simulink model "Simulink_model"  (Simulink 7.9)
settings: Solver=ode45  StartTime=0.0  StopTime=2  RelTol=1e-3
PreLoadFcn:
  | %% パラメータ設定
  | Ra = 1;%アーマチュア抵抗[Ω]
  | La = 1e-5;%アーマチュアインダクタンス[H]
  | KT = 0.05;%トルク定数[N*m/A]
  | KE = KT;%逆起定数[V*s/rad]
  | %その他パラメータ
  | K = 0.5;%バネ定数[N*m*rad^-1*s]
  | D = 5e-5;%粘性摩擦[N*m*rad^-1*s^2]
  | L = 0.02;%無駄時間[s]
  | 
  | JM = 1e-4;%ロータ側のイナーシャ[kg*m^2]
  | JL = 0.5e-4;%負荷側のイナーシャ[kg*m^2]
settings Model: Creator=hmita  LastModifiedBy=hmita
settings DebuggingCC: FcnCallInpInsideContextMsg=Use local settings
settings GRTTargetCC: CombineOutputUpdateFcns=off  GRTInterface=on

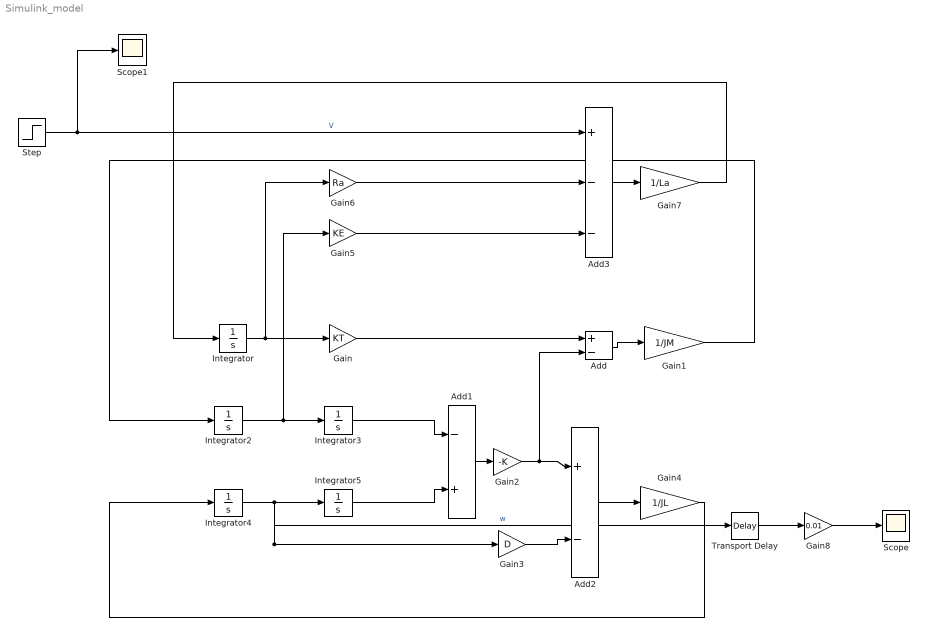
== system Simulink_model ==
  Add : Sum  Inputs=+-
  Add1 : Sum  Inputs=-+
  Add2 : Sum  Inputs=+-
  Add3 : Sum  Inputs=+--
  Gain : Gain  Gain=KT
  Gain1 : Gain  Gain=1/JM
  Gain2 : Gain  Gain=-K
  Gain3 : Gain  Gain=D
  Gain4 : Gain  Gain=1/JL
  Gain5 : Gain  Gain=KE
  Gain6 : Gain  Gain=Ra
  Gain7 : Gain  Gain=1/La
  Gain8 : Gain  Gain=0.01
  Integrator{,2..5} (5 alike) : Integrator
  Scope : Scope
  Scope1 : Scope
  Step : Step  SampleTime=0
  Transport Delay : TransportDelay  DelayTime=L
  wires:
  Integrator/1 -> Gain/1, Gain6/1
  Gain/1 -> Add/1
  Integrator2/1 -> Integrator3/1, Gain5/1
  Integrator3/1 -> Add1/1
  Gain7/1 -> Integrator/1
  Gain1/1 -> Integrator2/1
  Integrator5/1 -> Add1/2
  Integrator4/1 -> Integrator5/1, Gain3/1, Transport Delay/1  "w"
  Add/1 -> Gain1/1
  Add1/1 -> Gain2/1
  Gain2/1 -> Add/2, Add2/1
  Gain3/1 -> Add2/2
  Add2/1 -> Gain4/1
  Gain4/1 -> Integrator4/1
  Gain5/1 -> Add3/3
  Gain6/1 -> Add3/2
  Step/1 -> Add3/1, Scope1/1  "V"
  Add3/1 -> Gain7/1
  Transport Delay/1 -> Gain8/1
  Gain8/1 -> Scope/1
